simulink model "ADAS_system"  (R2025b)
settings: Solver=VariableStepAuto  StartTime=0.0  StopTime=10.0  RelTol=1e-3
values from neighbouring files (symbols this model uses):
  car_wheelbase = 2.0    (= 2)    [skrypt.m]
  max_steering_wheel = pi/6    (= 0.523598775598)    [skrypt.m]
undefined symbols (not defined in the file or in its folder): braking_threshold, distance_threshold, max_brake_when_slowing, warning_threshold
libraries: simulink x8, slpidlib x2
settings Model: Creator=julia  LastModifiedBy=mikir

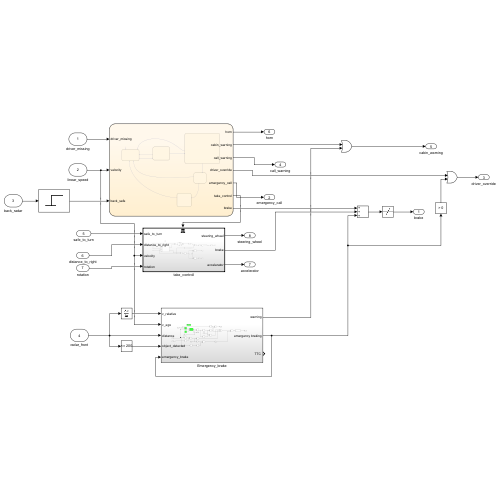
[thumbnail: Simulink's stored preview of the top-level diagram]
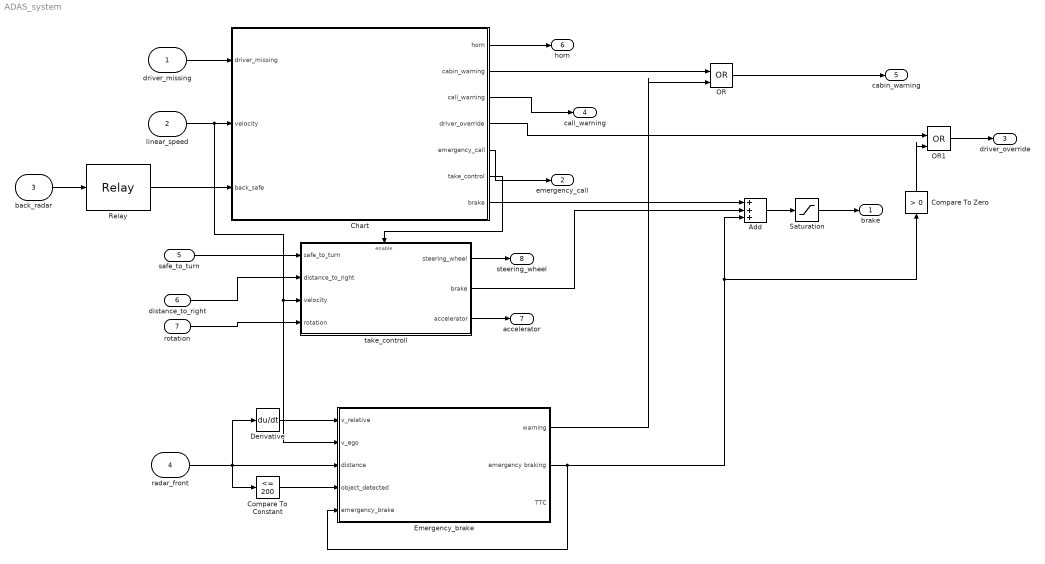
== system ADAS_system ==
  driver_missing : Inport
  linear_speed : Inport  Port=2
  back_radar : Inport  Port=3
  radar_front : Inport  Port=4
  safe_to_turn : Inport  Port=5
  distance_to_right : Inport  Port=6
  rotation : Inport  Port=7
  Add : Sum  Inputs=+++
  Chart : Stateflow chart  TreatAsAtomicUnit=on
  Compare To Constant : simulink/Logic and Bit Operations/Compare To Constant  relop=<=  const=200  OutDataTypeStr=boolean
  Compare To Zero : simulink/Logic and Bit Operations/Compare To Zero  relop=>  OutDataTypeStr=boolean
  Derivative : Derivative
  Emergency_brake : Subsystem
  OR : Logic  Operator=OR  IconShape=distinctive  AllPortsSameDT=off  OutDataTypeStr=boolean
  OR1 : Logic  Operator=OR  IconShape=distinctive  AllPortsSameDT=off  OutDataTypeStr=boolean
  Relay : Relay  OnSwitchValue=70  OffSwitchValue=60
  Saturation : Saturate  UpperLimit=1  LowerLimit=-1
  take_controll : Subsystem  TreatAsAtomicUnit=on
  brake : Outport
  emergency_call : Outport  Port=2
  driver_override : Outport  Port=3
  call_warning : Outport  Port=4
  cabin_warning : Outport  Port=5
  horn : Outport  Port=6
  accelerator : Outport  Port=7
  steering_wheel : Outport  Port=8
  wires:
  Relay/1 -> Chart/3(back_safe)
  back_radar/1 -> Relay/1
  Chart/3(call_warning) -> call_warning/1
  driver_missing/1 -> Chart/1(driver_missing)
  linear_speed/1 -> Emergency_brake/2(v_ego), take_controll/3(velocity), Chart/2(velocity)
  Chart/1(horn) -> horn/1
  distance_to_right/1 -> take_controll/2(distance_to_right)
  Chart/5(emergency_call) -> emergency_call/1
  Chart/6(take_control) -> take_controll/Enable
  Chart/7(brake) -> Add/1
  safe_to_turn/1 -> take_controll/1(safe_to_turn)
  rotation/1 -> take_controll/4(rotation)
  take_controll/1(steering_wheel) -> steering_wheel/1
  take_controll/2(brake) -> Add/2
  take_controll/3(accelerator) -> accelerator/1
  Add/1 -> Saturation/1
  Saturation/1 -> brake/1
  radar_front/1 -> Derivative/1, Compare To Constant/1, Emergency_brake/3(distance)
  Compare To Constant/1 -> Emergency_brake/4(object_detected)
  Derivative/1 -> Emergency_brake/1(v_relative)
  Emergency_brake/2(emergency braking) -> Emergency_brake/5(emergency_brake), Compare To Zero/1, Add/3
  Emergency_brake/1(warning) -> OR/2
  OR/1 -> cabin_warning/1
  OR1/1 -> driver_override/1
  Compare To Zero/1 -> OR1/2
  Chart/2(cabin_warning) -> OR/1
  Chart/4(driver_override) -> OR1/1

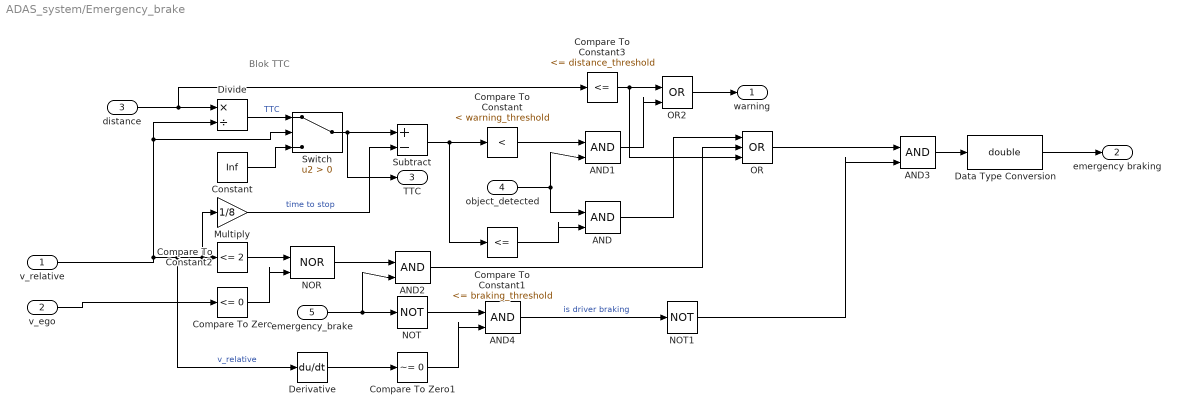
== system ADAS_system/Emergency_brake ==
  note: Blok TTC
  v_relative : Inport
  v_ego : Inport  Port=2
  distance : Inport  Port=3
  object_detected : Inport  Port=4
  emergency_brake : Inport  Port=5
  AND{,1..4} (5 alike) : Logic  IconShape=distinctive  AllPortsSameDT=off  OutDataTypeStr=boolean
  Compare To Constant : simulink/Logic and Bit Operations/Compare To Constant  relop=<  const=warning_threshold  OutDataTypeStr=boolean
  Compare To Constant1 : simulink/Logic and Bit Operations/Compare To Constant  relop=<=  const=braking_threshold  OutDataTypeStr=boolean
  Compare To Constant2 : simulink/Logic and Bit Operations/Compare To Constant  relop=<=  const=2  OutDataTypeStr=boolean
  Compare To Constant3 : simulink/Logic and Bit Operations/Compare To Constant  relop=<=  const=distance_threshold  OutDataTypeStr=boolean
  Compare To Zero : simulink/Logic and Bit Operations/Compare To Zero  relop=<=  OutDataTypeStr=boolean
  Compare To Zero1 : simulink/Logic and Bit Operations/Compare To Zero  relop=~=  OutDataTypeStr=boolean
  Constant : Constant  Value=Inf
  Data Type Conversion : DataTypeConversion  OutDataTypeStr=double  SaturateOnIntegerOverflow=off  RndMeth=Floor
  Derivative : Derivative
  Divide : Product  Inputs=*/
  Multiply : Gain  Gain=1/8
  NOR : Logic  Operator=NOR  IconShape=distinctive  AllPortsSameDT=off  OutDataTypeStr=boolean
  NOT : Logic  Operator=NOT  IconShape=distinctive  AllPortsSameDT=off  OutDataTypeStr=boolean
  NOT1 : Logic  Operator=NOT  IconShape=distinctive  AllPortsSameDT=off  OutDataTypeStr=boolean
  OR : Logic  Operator=OR  Inputs=3  IconShape=distinctive  AllPortsSameDT=off  OutDataTypeStr=boolean
  OR2 : Logic  Operator=OR  IconShape=distinctive  AllPortsSameDT=off  OutDataTypeStr=boolean
  Subtract : Sum  Inputs=+-
  Switch : Switch  Criteria=u2 > Threshold  SaturateOnIntegerOverflow=off  InputSameDT=off
  warning : Outport
  emergency braking : Outport  Port=2
  "TTC " : Outport  Port=3
  wires:
  Switch/1 -> "TTC "/1, Subtract/1
  Compare To Constant3/1 -> OR/3, OR2/1
  OR2/1 -> warning/1
  OR/1 -> AND3/1
  AND/1 -> OR/1
  v_relative/1 -> Multiply/1, Compare To Constant2/1, Derivative/1, Switch/2, Divide/2  "v_relative"
  AND2/1 -> OR/2
  Compare To Zero/1 -> NOR/2
  AND3/1 -> Data Type Conversion/1
  Compare To Zero1/1 -> AND4/2
  AND4/1 -> NOT1/1  "is driver braking"
  NOT/1 -> AND4/1
  AND1/1 -> OR2/2
  v_ego/1 -> Compare To Zero/1
  Derivative/1 -> Compare To Zero1/1
  Subtract/1 -> Compare To Constant1/1, Compare To Constant/1
  emergency_brake/1 -> NOT/1, AND2/2
  Divide/1 -> Switch/1  "TTC"
  distance/1 -> Compare To Constant3/1, Divide/1
  Compare To Constant/1 -> AND1/1
  object_detected/1 -> AND/1, AND1/2
  Multiply/1 -> Subtract/2  "time to stop"
  Constant/1 -> Switch/3
  Data Type Conversion/1 -> emergency braking/1
  Compare To Constant2/1 -> NOR/1
  NOT1/1 -> AND3/2
  Compare To Constant1/1 -> AND/2
  NOR/1 -> AND2/1

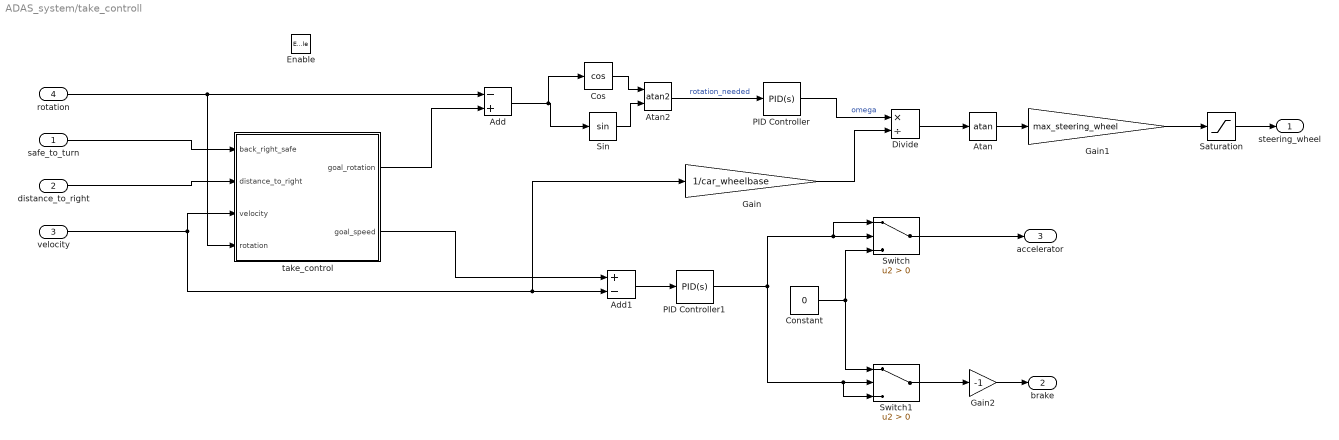
== system ADAS_system/take_controll ==
  safe_to_turn : Inport
  distance_to_right : Inport  Port=2
  velocity : Inport  Port=3
  rotation : Inport  Port=4
  Enable : EnablePort
  Add : Sum  Inputs=-+
  Add1 : Sum  Inputs=+-
  Atan : Trigonometry  Operator=atan
  Atan2 : Trigonometry  Operator=atan2
  Constant : Constant  Value=0
  Cos : Trigonometry  Operator=cos
  Divide : Product  Inputs=*/
  Gain : Gain  Gain=1/car_wheelbase
  Gain1 : Gain  Gain=max_steering_wheel
  Gain2 : Gain  Gain=-1
  PID Controller : slpidlib/PID Controller  Controller=PID  Form=Parallel  TimeDomain=Continuous-time  UseExternalTs=off  SampleTime=-1  IntegratorMethod=Forward Euler  FilterMethod=Forward Euler  ControllerParametersSource=internal  P=1  I=1  UseKiTs=off  D=0  UseExternalDerivativeSource=off  N=100  UseFilter=on  TunerSelectOption=Transfer Function Based (PID Tuner App)  InitialConditionSource=internal  InitialConditionForIntegrator=0  InitialConditionForFilter=0  DifferentiatorICPrevScaledInput=0  ExternalReset=none  TrackingMode=off  Kt=1  LimitOutput=off  SatLimitsSource=internal  UpperSaturationLimit=0.5  LowerSaturationLimit=-0.5  LinearizeAsGain=on  AntiWindupMode=none  Kb=1  LimitIntegrator=off  UpperIntegratorSaturationLimit=inf  LowerIntegratorSaturationLimit=-inf  POutMin=[]  POutMax=[]  IOutMin=[]  IOutMax=[]  DOutMin=[]  DOutMax=[]  NOutMin=[]  NOutMax=[]  SumOutMin=[]  SumOutMax=[]  SaturationOutMin=[]  SaturationOutMax=[]  PParamMin=[]  PParamMax=[]  IParamMin=[]  IParamMax=[]  DParamMin=[]  DParamMax=[]  NParamMin=[]  NParamMax=[]  KbParamMin=[]  KbParamMax=[]  KtParamMin=[]  KtParamMax=[]  KbOutMin=[]  KbOutMax=[]  KtOutMin=[]  KtOutMax=[]  IntegratorOutMin=[]  IntegratorOutMax=[]  FilterOutMin=[]  FilterOutMax=[]  SumI1OutMin=[]  SumI1OutMax=[]  SumI2OutMin=[]  SumI2OutMax=[]  SumI3OutMin=[]  SumI3OutMax=[]  SumI4OutMin=[]  SumI4OutMax=[]  SumDOutMin=[]  SumDOutMax=[]  DifferentiatorOutMin=[]  DifferentiatorOutMax=[]  FilterDiffOutCoefMin=[]  FilterDiffOutCoefMax=[]  ReciprocalOutMin=[]  ReciprocalOutMax=[]  SumDenOutMin=[]  SumDenOutMax=[]  SumNumOutMin=[]  SumNumOutMax=[]  DivideOutMin=[]  DivideOutMax=[]  UdiffTsProdOutMin=[]  UdiffTsProdOutMax=[]  NTsProdOutMin=[]  NTsProdOutMax=[]  UintegralTsProdOutMin=[]  UintegralTsProdOutMax=[]  UngainTsProdOutMin=[]  UngainTsProdOutMax=[]  ClampingZeroOutDataTypeStr=Inherit: Inherit via back propagation  ClampingZeroOutMin=[]  ClampingZeroOutMax=[]  FilterDenConstantOutDataTypeStr=Inherit: Inherit via back propagation  FilterDenConstantOutMin=[]  FilterDenConstantOutMax=[]  PCopyOutDataTypeStr=Inherit: Inherit via back propagation  PCopyOutMin=[]  PCopyOutMax=[]  NCopyOutDataTypeStr=Inherit: Inherit via back propagation  NCopyOutMin=[]  NCopyOutMax=[]  IntegratorContinuousStateAttributes=''  IntegratorStateMustResolveToSignalObject=off  IntegratorRTWStateStorageClass=Auto  FilterContinuousStateAttributes=''  FilterStateMustResolveToSignalObject=off  FilterRTWStateStorageClass=Auto  ParallelPVariant=InternalParameters  IdealPVariant=Disabled  IVariant=InternalParameters  DVariant=InternalParameters  IntegratorVariant=Continuous  SatVariant=Disabled  AWVariant=Passthrough  PCopyVariant=Disabled  TRVariant=Disabled  FdbkBlocksVariant=Forward  IdealPFdbkVariant=Disabled  SatFdbkVariant=Disabled  DerivativeFilterVariant=ContFilter  NVariant=InternalParameters  NCopyVariant=Disabled  FilterICVariant=InternalICsFilter  IntegratorICVariant=InternalICs  ExternalResetVariant=Disabled  TRSumVariant=Passthrough  SumFdbkVariant=Disabled  SumVariant=Sum_PID  TsampFilterVariant=InternalTs  TsampNgainVariant=Passthrough  TsampIntegralVariant=Disabled_SignalSpec  ExternalSaturationOutDataTypeStr=Inherit: Same as second input  DerivativeSourceVariant=ErrorSignal  PreIntVariant=InternalPreInt
  PID Controller1 : slpidlib/PID Controller  Controller=PID  Form=Parallel  TimeDomain=Continuous-time  UseExternalTs=off  SampleTime=-1  IntegratorMethod=Forward Euler  FilterMethod=Forward Euler  ControllerParametersSource=internal  P=1  I=1  UseKiTs=off  D=0  UseExternalDerivativeSource=off  N=100  UseFilter=on  TunerSelectOption=Transfer Function Based (PID Tuner App)  InitialConditionSource=internal  InitialConditionForIntegrator=0  InitialConditionForFilter=0  DifferentiatorICPrevScaledInput=0  ExternalReset=none  TrackingMode=off  Kt=1  LimitOutput=on  SatLimitsSource=internal  UpperSaturationLimit=max_brake_when_slowing  LowerSaturationLimit=-max_brake_when_slowing  LinearizeAsGain=on  AntiWindupMode=none  Kb=1  LimitIntegrator=off  UpperIntegratorSaturationLimit=inf  LowerIntegratorSaturationLimit=-inf  POutMin=[]  POutMax=[]  IOutMin=[]  IOutMax=[]  DOutMin=[]  DOutMax=[]  NOutMin=[]  NOutMax=[]  SumOutMin=[]  SumOutMax=[]  SaturationOutMin=[]  SaturationOutMax=[]  PParamMin=[]  PParamMax=[]  IParamMin=[]  IParamMax=[]  DParamMin=[]  DParamMax=[]  NParamMin=[]  NParamMax=[]  KbParamMin=[]  KbParamMax=[]  KtParamMin=[]  KtParamMax=[]  KbOutMin=[]  KbOutMax=[]  KtOutMin=[]  KtOutMax=[]  IntegratorOutMin=[]  IntegratorOutMax=[]  FilterOutMin=[]  FilterOutMax=[]  SumI1OutMin=[]  SumI1OutMax=[]  SumI2OutMin=[]  SumI2OutMax=[]  SumI3OutMin=[]  SumI3OutMax=[]  SumI4OutMin=[]  SumI4OutMax=[]  SumDOutMin=[]  SumDOutMax=[]  DifferentiatorOutMin=[]  DifferentiatorOutMax=[]  FilterDiffOutCoefMin=[]  FilterDiffOutCoefMax=[]  ReciprocalOutMin=[]  ReciprocalOutMax=[]  SumDenOutMin=[]  SumDenOutMax=[]  SumNumOutMin=[]  SumNumOutMax=[]  DivideOutMin=[]  DivideOutMax=[]  UdiffTsProdOutMin=[]  UdiffTsProdOutMax=[]  NTsProdOutMin=[]  NTsProdOutMax=[]  UintegralTsProdOutMin=[]  UintegralTsProdOutMax=[]  UngainTsProdOutMin=[]  UngainTsProdOutMax=[]  ClampingZeroOutDataTypeStr=Inherit: Inherit via back propagation  ClampingZeroOutMin=[]  ClampingZeroOutMax=[]  FilterDenConstantOutDataTypeStr=Inherit: Inherit via back propagation  FilterDenConstantOutMin=[]  FilterDenConstantOutMax=[]  PCopyOutDataTypeStr=Inherit: Inherit via back propagation  PCopyOutMin=[]  PCopyOutMax=[]  NCopyOutDataTypeStr=Inherit: Inherit via back propagation  NCopyOutMin=[]  NCopyOutMax=[]  IntegratorContinuousStateAttributes=''  IntegratorStateMustResolveToSignalObject=off  IntegratorRTWStateStorageClass=Auto  FilterContinuousStateAttributes=''  FilterStateMustResolveToSignalObject=off  FilterRTWStateStorageClass=Auto  ParallelPVariant=InternalParameters  IdealPVariant=Disabled  IVariant=InternalParameters  DVariant=InternalParameters  IntegratorVariant=Continuous  SatVariant=Enabled  AWVariant=Passthrough  PCopyVariant=Disabled  TRVariant=Disabled  FdbkBlocksVariant=Forward  IdealPFdbkVariant=Disabled  SatFdbkVariant=Disabled  DerivativeFilterVariant=ContFilter  NVariant=InternalParameters  NCopyVariant=Disabled  FilterICVariant=InternalICsFilter  IntegratorICVariant=InternalICs  ExternalResetVariant=Disabled  TRSumVariant=Passthrough  SumFdbkVariant=Disabled  SumVariant=Sum_PID  TsampFilterVariant=InternalTs  TsampNgainVariant=Passthrough  TsampIntegralVariant=Disabled_SignalSpec  ExternalSaturationOutDataTypeStr=Inherit: Same as second input  DerivativeSourceVariant=ErrorSignal  PreIntVariant=InternalPreInt
  Saturation : Saturate
  Sin : Trigonometry
  Switch : Switch  Criteria=u2 > Threshold  SaturateOnIntegerOverflow=off  InputSameDT=off
  Switch1 : Switch  Criteria=u2 > Threshold  SaturateOnIntegerOverflow=off  InputSameDT=off
  take_control : Stateflow chart  TreatAsAtomicUnit=on
  steering_wheel : Outport
  brake : Outport  Port=2
  accelerator : Outport  Port=3
  wires:
  distance_to_right/1 -> take_control/2(distance_to_right)
  safe_to_turn/1 -> take_control/1(back_right_safe)
  velocity/1 -> Gain/1, Add1/2, take_control/3(velocity)
  take_control/1(goal_rotation) -> Add/2
  rotation/1 -> take_control/4(rotation), Add/1
  Add/1 -> Sin/1, Cos/1
  Sin/1 -> Atan2/2
  Cos/1 -> Atan2/1
  Atan2/1 -> PID Controller/1  "rotation_needed"
  PID Controller/1 -> Divide/1  "omega"
  Gain/1 -> Divide/2
  Divide/1 -> Atan/1
  Atan/1 -> Gain1/1
  Gain1/1 -> Saturation/1
  Saturation/1 -> steering_wheel/1
  take_control/2(goal_speed) -> Add1/1
  Add1/1 -> PID Controller1/1
  PID Controller1/1 -> Switch/1, Switch/2, Switch1/3, Switch1/2
  Constant/1 -> Switch1/1, Switch/3
  Switch/1 -> accelerator/1
  Switch1/1 -> Gain2/1
  Gain2/1 -> brake/1

== stateflow chart ADAS_system/take_controll/take_control ==
  state waiting_for_space
    en:
    goal_speed = 0;
    ex:
    goal_speed = speed_when_pulling_over;
  state slowing_down
    en:
    goal_speed = speed_when_pulling_over;
  state pulling_over
    en:
    goal_rotation = rotation_when_pulling_over;
  state positioning
    en:
    goal_rotation=0
    goal_speed =2
  state stopping
    en:
    goal_speed=0;
  slowing_down -> waiting_for_space : [velocity == speed_when_pulling_over]
  waiting_for_space -> pulling_over : [back_right_safe]
  pulling_over -> waiting_for_space [order 2] : [~back_right_safe]
  (default) -> slowing_down
  pulling_over -> positioning [order 1] : [distance_to_right<1]
  positioning -> stopping : [rotation==0]
  data: back_right_safe input; distance_to_right input; velocity input; goal_rotation output; rotation_when_pulling_over constant double; speed_when_pulling_over constant double; goal_speed output; rotation input

== stateflow chart ADAS_system/Chart ==
  state warning_phase_2
    en:
    cabin_warning = true;
    horn = false;
    brake = 0;
    du:
    if (temporalCount(sec) < 1)
    horn = true;
    else
    horn = false;
    end
    if (back_safe == true && temporalCount(sec) >1 && temporalCount(sec) < 1.3)
    driver_override = true;
    brake = 1;
    else
    brake = 0;
    driver_override = false;
    end
    ex:
    brake = 0;
    horn = false;
    cabin_warning = false;
  state warning_phase_1
    en:
    cabin_warning = true;
    ex:
    cabin_warning = false;
  state do_nothing
    en:
    cabin_warning = false;
    driver_override =false;
  state take_control
    en:
    driver_override = true;
    take_control = true;
    ex:
    take_control = false;
    driver_override = false;
  state emergency_stop
    en:
    call_warning = true;
    du:
    if (temporalCount(sec) > 5)
    emergency_call = true
    end
    ex:
    call_warning = false;
    emergency_call = false;
  warning_phase_2 -> do_nothing [order 2] : [driver_missing==false]
  (default) -> do_nothing
  warning_phase_1 -> warning_phase_2 [order 2] : [after(1,sec)]
  warning_phase_1 -> do_nothing [order 1] : [driver_missing==false]
  do_nothing -> warning_phase_1 : [driver_missing==1]
  emergency_stop -> do_nothing : [driver_missing==false]
  take_control -> do_nothing [order 2] : [driver_missing==false]
  warning_phase_2 -> take_control [order 1] : [after(2,sec)]
  take_control -> emergency_stop [order 1] : [velocity == 0]
  data: driver_missing input; horn output; cabin_warning output; velocity input; back_safe input; call_warning output; driver_override output; emergency_call output; take_control output; brake output
